simulink model "UARTReadLine2"  (R2017b)
settings: Solver=FixedStepDiscrete  StartTime=0.0  StopTime=10.0  FixedStep=1e-3  RelTol=1e-3
libraries: mbed_lib x5
settings Model: Creator=oh  LastModifiedBy=oh
settings DataIOCC: LimitDataPoints=on  SaveFormat=Array
settings OptimizationCC: LifeSpan=1
settings DebuggingCC: SFUnexpectedBacktrackingDiag=warning  SFNoUnconditionalDefaultTransitionDiag=warning  SFExecutionAtInitializationDiag=none
settings HardwareCC: ProdBitPerPointer=32  ProdBitPerSizeT=32  ProdBitPerPtrDiffT=32  ProdLargestAtomicInteger=Long  ProdLargestAtomicFloat=Double  ProdIntDivRoundTo=Undefined  ProdWordSize=32  ProdHWDeviceType=ARM Compatible->ARM Cortex
settings ModelReferenceCC: PropagateSignalLabelsOutOfModel=off
settings SFSimCC: MATLABDynamicMemAlloc=off
settings RTWCC: SystemTargetFile=mbed.tlc  TemplateMakefile=mbed.tmf  Description=Mbed Target (Embedded Target)  TargetLang=C++
settings CodeAppCC: IgnoreCustomStorageClasses=off  StateflowObjectComments=on
settings STFCustomTargetCC: TargetLibSuffix=.a  GenerateSampleERTMain=on  CombineOutputUpdateFcns=on  ERTCustomFileBanners=on  SupportContinuousTime=off  SupportNonInlinedSFcns=off  RemoveResetFunc=on  SupportVariableSizeSignals=on  MATLABClassNameForMDSCustomization=Simulink.SoftwareTarget.ERTCustomization  ModelStepFunctionPrototypeControlCompliant=on  GRTInterface=off  SystemTargetFile=mbed.tlc
settings ERTTargetCC: MultiwordLength=2048  GenerateSampleERTMain=on  ParMdlRefBuildCompliant=off  CompOptLevelCompliant=off  ConcurrentExecutionCompliant=off  SupportVariableSizeSignals=on  CPPClassGenCompliant=off  UseToolchainInfoCompliant=off  ERTCustomFileTemplate=mbed_file_process.tlc  ConvertIfToSwitch=off  SuppressUnreachableDefaultCases=off
settings ConfigComp: CovMetricSettings=dw  CovHtmlReporting=on  CovSaveCumulativeToWorkspaceVar=on  CovSaveSingleToWorkspaceVar=on  CovExternalEMLEnable=off

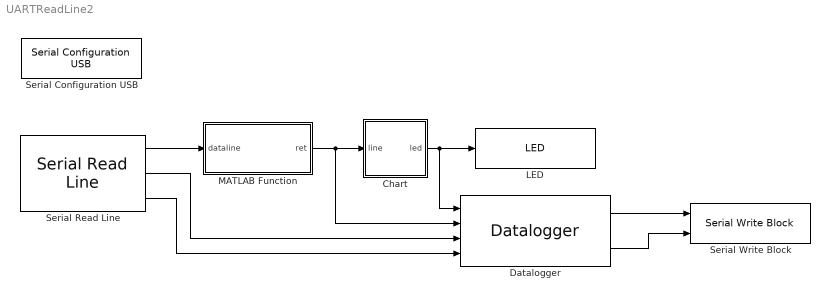
== system UARTReadLine2 ==
  Chart : Stateflow chart  TreatAsAtomicUnit=on
  Datalogger : mbed_lib/Utilities/Datalogger  TypeInputPorts={ 'uint8' 1 'uint8' 1 'uint32' 1 'uint8' 1 }  TypeOfInputs={'1*uint8' '1*uint8' '1*uint32' '1*uint8'}  BufferSize=10  errEn=off  SampleTime=-1
      settings: SourceProductName=Mbed Target
  LED : mbed_lib/GPIO/LED  nLED=1  SampleTime=-1
      settings: SourceProductName=Mbed Target
  MATLAB Function : MATLAB Function  TreatAsAtomicUnit=on
  Serial Configuration USB : mbed_lib/Serial/UART/Serial Configuration USB  Priority=0  BaudRate=9600
      settings: AttributesFormatString=%<Priority>=10  SourceProductName=Mbed Target
  Serial Read Line : mbed_lib/Serial/UART/Serial Read Line  SerialPort=USB  NumDataPort=on  NewDataPort=on  BufferSize=5  SampleTime=0.5
      settings: SourceProductName=Mbed Target
  Serial Write Block : mbed_lib/Serial/UART/Serial Write Block  SerialPort=USB  numData=on  SampleTime=-1
      settings: SourceProductName=Mbed Target
  wires:
  Serial Read Line/3 -> Datalogger/4
  Serial Read Line/2 -> Datalogger/3
  Chart/1(led) -> Datalogger/1, LED/1
  MATLAB Function/1(ret) -> Datalogger/2, Chart/1(line)
  Serial Read Line/1 -> MATLAB Function/1(dataline)
  Datalogger/1 -> Serial Write Block/1
  Datalogger/2 -> Serial Write Block/2

== matlab function UARTReadLine2/MATLAB Function ==
  data: ret output; dataline input
function ret = strmulticompare(dataline)

commands = {'on', 'off'};
ret = uint8(0);

for i=1:size(commands,2)
    ok=uint8(1);
    for j=1:size(commands{i},2)
        if commands{i}(j)~=dataline(j)
            ok=uint8(0);
            break;
        end
    end
    if ok==uint8(1)
      ret = uint8(i);
      return;
    end
end

== stateflow chart UARTReadLine2/Chart ==
  state start
  (default) -> start
  start -> start [order 1] : [line==uint8(1)]{led=1;}
  start -> start [order 2] : [line==uint8(2)]{led=0;}
  data: line input; led output uint8
